simulink model "Position"  (R2022a)
settings: Solver=ode1  StartTime=0.0  StopTime=inf  FixedStep=0.01  RelTol=1e-3  EnableMultiTasking=on
undefined symbols (not defined in the file): a, b, k1, k2, kd4, kp4
libraries: arduinolib x6, arduinosensorlib x2, simulink_extras x2
settings Model: ExtModeTrigDuration=2  Creator=LabPC  LastModifiedBy=LabPC
settings OptimizationCC: EnhancedBackFolding=on  PassReuseOutputArgsAs=Individual arguments  ZeroExternalMemoryAtStartup=off  ZeroInternalMemoryAtStartup=off  MaxStackSize=64  OptimizeBlockOrder=speed  DifferentSizesBufferReuse=on  OptimizationCustomize=off  EfficientTunableParamExpr=on
settings DebuggingCC: ParameterTunabilityLossMsg=error
settings HardwareCC: ProdBitPerInt=16  ProdBitPerPointer=16  ProdBitPerSizeT=16  ProdBitPerPtrDiffT=16  ProdLargestAtomicFloat=None  ProdWordSize=8  ProdHWDeviceType=Atmel->AVR
settings SFSimCC: MATLABDynamicMemAlloc=off
settings RTWCC: SystemTargetFile=ert.tlc  HardwareBoard=Arduino Mega 2560  TemplateMakefile=ert_default_tmf  Toolchain=Arduino AVR  BuildConfiguration=Faster Runs
settings CodeAppCC: ForceParamTrailComments=on  IgnoreCustomStorageClasses=off  OperatorAnnotations=on  SimulinkDataObjDesc=on  SFDataObjDesc=on  InsertBlockDesc=on
settings ERTTargetCC: SupportContinuousTime=on  SupportVariableSizeSignals=on  ExtModeTransport=3  ExtModeStaticAlloc=on  ExtModeStaticAllocSize=2048  ExtModeMexFile=ext_xcp  ExtModeIntrfLevel=Level2 - Open

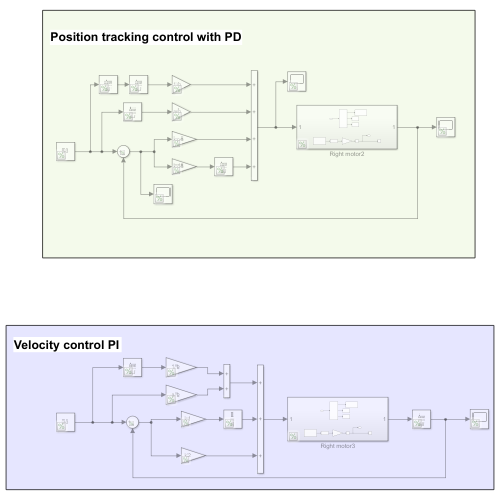
[thumbnail: Simulink's stored preview of the top-level diagram]
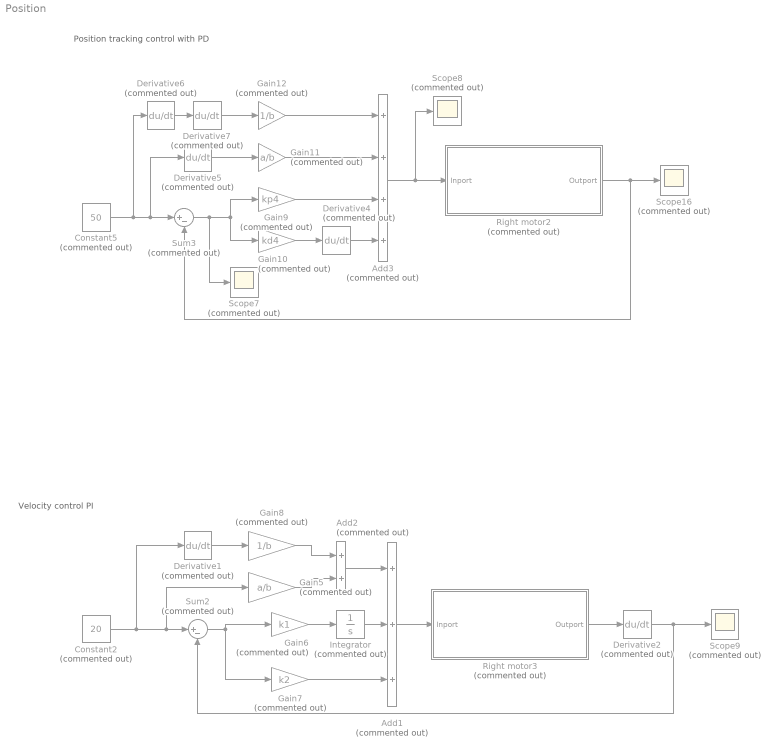
== system Position ==
  note: Position tracking control with PD
  note: Velocity control PI
  Add1 : Sum  Commented=on  Inputs=+++
  Add2 : Sum  Commented=on
  Add3 : Sum  Commented=on  Inputs=++++
  Constant2 : Constant  Commented=on  Value=20
  Constant5 : Constant  Commented=on  Value=50
  Derivative{1..2,4..7} (6 alike) : Derivative  Commented=on
  Gain10 : Gain  Commented=on  Gain=kd4
  Gain11 : Gain  Commented=on  Gain=a/b
  Gain12 : Gain  Commented=on  Gain=1/b
  Gain5 : Gain  Commented=on  Gain=a/b
  Gain6 : Gain  Commented=on  Gain=k1
  Gain7 : Gain  Commented=on  Gain=k2
  Gain8 : Gain  Commented=on  Gain=1/b
  Gain9 : Gain  Commented=on  Gain=kp4
  Integrator : Integrator  Commented=on
  Right motor2 : Subsystem  Commented=on
  Right motor3 : Subsystem  Commented=on
  Scope{7..9,16} (4 alike) : Scope  Commented=on
  Sum2 : Sum  Commented=on  Inputs=|+-
  Sum3 : Sum  Commented=on  Inputs=|+-
  wires:
  Derivative7/1 -> Gain12/1
  Gain9/1 -> Add3/3
  Gain12/1 -> Add3/1
  Gain11/1 -> Add3/2
  Sum3/1 -> Scope7/1, Gain9/1, Gain10/1
  Derivative5/1 -> Gain11/1
  Derivative6/1 -> Derivative7/1
  Add3/1 -> Scope8/1, Right motor2/1(Inport)
  Constant5/1 -> Derivative6/1, Derivative5/1, Sum3/1
  Gain10/1 -> Derivative4/1
  Derivative4/1 -> Add3/4
  Right motor2/1(Outport) -> Sum3/2, Scope16/1
  Sum2/1 -> Gain6/1, Gain7/1
  Integrator/1 -> Add1/2
  Gain6/1 -> Integrator/1
  Gain7/1 -> Add1/3
  Gain8/1 -> Add2/1
  Add2/1 -> Add1/1
  Derivative2/1 -> Scope9/1, Sum2/2
  Right motor3/1(Outport) -> Derivative2/1
  Add1/1 -> Right motor3/1(Inport)
  Gain5/1 -> Add2/2
  Constant2/1 -> Gain5/1, Sum2/1, Derivative1/1
  Derivative1/1 -> Gain8/1

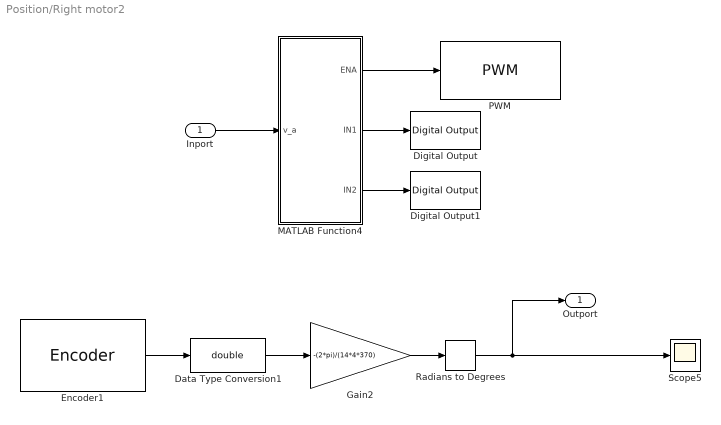
== system Position/Right motor2 ==
  Inport : Inport
  Data Type Conversion1 : DataTypeConversion  OutDataTypeStr=double  SaturateOnIntegerOverflow=off  RndMeth=Floor
  Digital Output : arduinolib/Digital Output  pinNumber=5  Direction=output  blockPlatform=arduino
  Digital Output1 : arduinolib/Digital Output  pinNumber=7  Direction=output  blockPlatform=arduino
  Encoder1 : arduinosensorlib/Encoder  InputA=2  InputB=3  Mode=No reset  SampleTime=-1
      settings: SourceProductBaseCode=ARDUINO
  Gain2 : Gain  Gain=-(2*pi)/(14*4*370)
  MATLAB Function4 : MATLAB Function  TreatAsAtomicUnit=on
  PWM : arduinolib/PWM  pinNumber=4  frequencyType=Default  desiredFrequency=490.2  achievableFrequency=490.2
  Radians to Degrees : simulink_extras/Transformations/Radians to Degrees
  Scope5 : Scope
  Outport : Outport
  wires:
  Gain2/1 -> Radians to Degrees/1
  Data Type Conversion1/1 -> Gain2/1
  Encoder1/1 -> Data Type Conversion1/1
  MATLAB Function4/1(ENA) -> PWM/1
  MATLAB Function4/2(IN1) -> Digital Output/1
  MATLAB Function4/3(IN2) -> Digital Output1/1
  Inport/1 -> MATLAB Function4/1(v_a)
  Radians to Degrees/1 -> Outport/1, Scope5/1

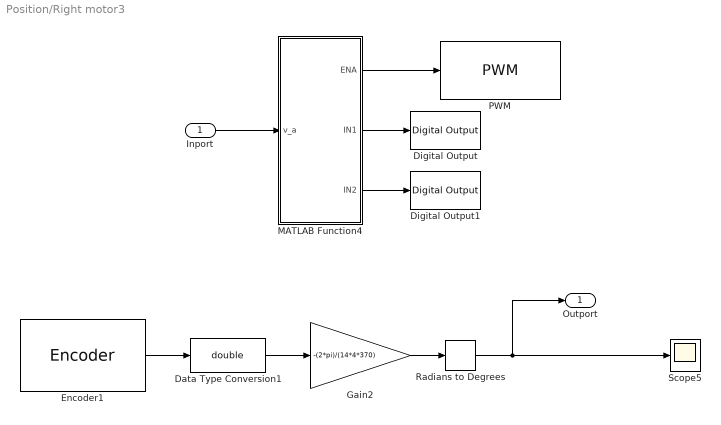
== system Position/Right motor3 ==
  Inport : Inport
  Data Type Conversion1 : DataTypeConversion  OutDataTypeStr=double  SaturateOnIntegerOverflow=off  RndMeth=Floor
  Digital Output : arduinolib/Digital Output  pinNumber=5  Direction=output  blockPlatform=arduino
  Digital Output1 : arduinolib/Digital Output  pinNumber=7  Direction=output  blockPlatform=arduino
  Encoder1 : arduinosensorlib/Encoder  InputA=2  InputB=3  Mode=No reset  SampleTime=-1
      settings: SourceProductBaseCode=ARDUINO
  Gain2 : Gain  Gain=-(2*pi)/(14*4*370)
  MATLAB Function4 : MATLAB Function  TreatAsAtomicUnit=on
  PWM : arduinolib/PWM  pinNumber=4  frequencyType=Default  desiredFrequency=490.2  achievableFrequency=490.2
  Radians to Degrees : simulink_extras/Transformations/Radians to Degrees
  Scope5 : Scope
  Outport : Outport
  wires:
  Radians to Degrees/1 -> Scope5/1, Outport/1
  Inport/1 -> MATLAB Function4/1(v_a)
  MATLAB Function4/3(IN2) -> Digital Output1/1
  MATLAB Function4/2(IN1) -> Digital Output/1
  MATLAB Function4/1(ENA) -> PWM/1
  Encoder1/1 -> Data Type Conversion1/1
  Data Type Conversion1/1 -> Gain2/1
  Gain2/1 -> Radians to Degrees/1

== matlab function Position/Right motor3/MATLAB Function4 ==
  data: v_a input; ENA output; IN1 output; IN2 output
function [ENA,IN1,IN2] = fcn(v_a)

vmax = 12;
pwm_cal = v_a*254/vmax;

if pwm_cal > 0
   
    ENA = pwm_cal;
    IN1 = 1;
    IN2 = 0;
elseif pwm_cal < 0
   
    ENA = abs(pwm_cal);
    IN1 = 0;
    IN2 = 1;
else
    ENA = 0;
    IN1 = 0;
    IN2 = 0;
   
end

== matlab function Position/Right motor2/MATLAB Function4 ==
  data: v_a input; ENA output; IN1 output; IN2 output
function [ENA,IN1,IN2] = fcn(v_a)

vmax = 12;
pwm_cal = v_a*254/vmax;

if pwm_cal > 0
   
    ENA = pwm_cal;
    IN1 = 1;
    IN2 = 0;
elseif pwm_cal < 0
   
    ENA = abs(pwm_cal);
    IN1 = 0;
    IN2 = 1;
else
    ENA = 0;
    IN1 = 0;
    IN2 = 0;
   
end
